simulink model "Integration_Backward_Forger_L"  (R2015a)
settings: Solver=ode3  StartTime=0.0  StopTime=T_opt  FixedStep=0.01  MaxStep=0.01  RelTol=1e-3
values from neighbouring files (symbols this model uses):
  R1_final = -(x(end,2)-xr_final)/((x(end,2)-xr_final)*(dx_final-dxr)+(xc(end,2)-xcr_final)*(dxc_final-dxcr))    [Gradient_Descent_Greedy_3rd.m]
  R2_final = -(xc(end,2)-xcr_final)/((x(end,2)-xr_final)*(dx_final-dxr)+(xc(end,2)-xcr_final)*(dxc_final-dxcr))    [Gradient_Descent_Greedy_3rd.m]
  R3_final = 0    [Gradient_Descent_Greedy_3rd.m]
  T_opt = x(end,1)    [Gradient_Descent_Greedy_3rd.m]
undefined symbols (not defined in the file or in its folder): I, x, xc
settings Model: Creator=wangf7  LastModifiedBy=Jiawei Yin
settings OptimizationCC: ExpressionDepthLimit=2147483647
settings DebuggingCC: UnderspecifiedInitializationDetection=Classic  MergeDetectMultiDrivingBlocksExec=none  SolverPrmCheckMsg=warning  StateNameClashWarn=warning

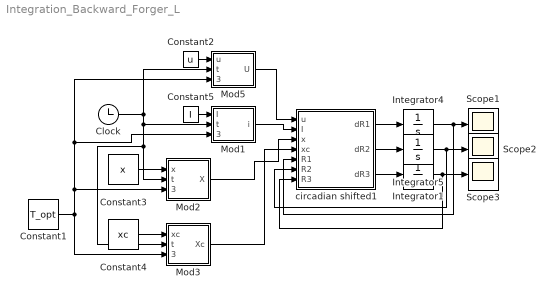
== system Integration_Backward_Forger_L ==
  Clock : Clock
  Constant1 : Constant  Value=T_opt
  Constant2 : Constant  Value=u
  Constant3 : Constant  Value=x
  Constant4 : Constant  Value=xc
  Constant5 : Constant  Value=I
  Integrator1 : Integrator  InitialCondition=R3_final
  Integrator4 : Integrator  InitialCondition=R1_final
  Integrator5 : Integrator  InitialCondition=R2_final
  Mod1 : MATLAB Function  TreatAsAtomicUnit=on
      settings: PermitHierarchicalResolution=ParametersOnly
  Mod2 : MATLAB Function  TreatAsAtomicUnit=on
      settings: PermitHierarchicalResolution=ParametersOnly
  Mod3 : MATLAB Function  TreatAsAtomicUnit=on
      settings: PermitHierarchicalResolution=ParametersOnly
  Mod5 : MATLAB Function  TreatAsAtomicUnit=on
      settings: PermitHierarchicalResolution=ParametersOnly
  Scope1 : Scope
      settings: TimeRange=auto  LimitDataPoints=on  MaxDataPoints=50000000  SaveName=R1  YMin=-0.12715  YMax=0.13151  SampleTime=-1  DataFormat=Array
  Scope2 : Scope
      settings: TimeRange=auto  LimitDataPoints=on  MaxDataPoints=50000000  SaveName=R2  YMin=-0.12825  YMax=0.13002  SampleTime=-1  DataFormat=Array
  Scope3 : Scope
      settings: TimeRange=auto  LimitDataPoints=on  MaxDataPoints=50000000  SaveName=R3  YMin=-0.12825  YMax=0.13002  SampleTime=-1  DataFormat=Array
  circadian shifted1 : MATLAB Function  TreatAsAtomicUnit=on
      settings: PermitHierarchicalResolution=ParametersOnly
  wires:
  circadian shifted1/1(dR1) -> Integrator4/1
  circadian shifted1/2(dR2) -> Integrator5/1
  Integrator4/1 -> circadian shifted1/5(R1), Scope1/1
  Integrator5/1 -> circadian shifted1/6(R2), Scope2/1
  Clock/1 -> Mod1/2(t), Mod2/2(t), Mod3/2(t), Mod5/2(t)
  Constant1/1 -> Mod3/3(T_opt), Mod5/3(T_opt), Mod1/3(T_opt), Mod2/3(T_opt)
  Mod2/1(X) -> circadian shifted1/3(x)
  Constant3/1 -> Mod2/1(x)
  Constant4/1 -> Mod3/1(xc)
  Mod3/1(Xc) -> circadian shifted1/4(xc)
  Constant5/1 -> Mod1/1(I)
  Mod1/1(i) -> circadian shifted1/2(I)
  Constant2/1 -> Mod5/1(u)
  Mod5/1(U) -> circadian shifted1/1(u)
  circadian shifted1/3(dR3) -> Integrator1/1
  Integrator1/1 -> circadian shifted1/7(R3), Scope3/1

== matlab function Integration_Backward_Forger_L/Mod2 ==
  data: x input; X output; t input; T_opt input
function X  = fcn(x,t,T_opt)
%#codegen
X=interp1q(x(:,1),x(:,2),T_opt-t);

== matlab function Integration_Backward_Forger_L/Mod1 ==
  data: I input; i output; t input; T_opt input
function i  = fcn(I,t,T_opt)
%#codegen
i=interp1q(I(:,1),I(:,2),T_opt-t);

== matlab function Integration_Backward_Forger_L/circadian shifted1 ==
  data: u input; I input; x input; xc input; dR1 output; R1 input; R2 input; dR2 output; R3 input; dR3 output
function [dR1,dR2,dR3] = fcn(u,I,x,xc,R1,R2,R3)

k=0.55;
mu=0.13;
q=1/3;
%B=(1-0.4*x)*(1-0.4*xc)*u;
tau=24.2;
I0=9500;
G=33.75;
p=0.5;
alpha0=0.05;
beta=0.0075;
% dx = pi*(xc+mu*(x/3+4*x^3/3-256*x^7/105)+B)/12;
% dxc = pi*(q*B*xc-x*((24/0.99729/tau)^2+k*B))/12;
dR1 = pi*R1*(mu*(1/3+4*x^2-256*x^6/15)-0.4*(1-0.4*xc)*u)/12+pi*R2*(-0.4*q*(1-0.4*xc)*xc*u-(24/0.99729/tau)^2-k*(1-0.8*x)*(1-0.4*xc)*u)/12;
dR2 = pi*R1*(1-0.4*(1-0.4*x)*u)/12+pi*R2*(q*(1-0.4*x)*(1-0.8*xc)*u+0.4*k*x*(1-0.4*x)*u)/12;
dR3 = -pi*R1*G*alpha0*(I/I0)^p*(1-0.4*x)*(1-0.4*xc)/12-pi*R2*(q*xc-k*x)*G*alpha0*(I/I0)^p*(1-0.4*x)*(1-0.4*xc)/12-60*R3*(alpha0*(I/I0)^p+beta);

== matlab function Integration_Backward_Forger_L/Mod3 ==
  data: xc input; Xc output; t input; T_opt input
function Xc  = fcn(xc,t,T_opt)
%#codegen
Xc=interp1q(xc(:,1),xc(:,2),T_opt-t);

== matlab function Integration_Backward_Forger_L/Mod5 ==
  data: u input; U output; t input; T_opt input
function U  = fcn(u,t,T_opt)
%#codegen
U=interp1q(u(:,1),u(:,2),T_opt-t);
